simulink model "IP_with_error"  (R2016b)
settings: Solver=FixedStepAuto  StartTime=0.0  StopTime=100  RelTol=1e-3  EnableMultiTasking=on
values from neighbouring files (symbols this model uses):
  A = [0 0 1 0 ... (first row only)    [Controller_IP_with_error.m]    (also in Controller_IP_without_error.m)
  B = [0;0;1;3]    [Controller_IP_with_error.m]    (also in Controller_IP_without_error.m)
  Bw = [0.0015;0.007;0.075;0.35]    [Controller_IP_with_error.m]    (also in Controller_IP_without_error.m)
  K = Ymat*inv(Xmat)    [Controller_IP_with_error.m]    (also in Controller_IP_without_error.m)
settings Model: Creator=Li  LastModifiedBy=silen
settings DataIOCC: LimitDataPoints=on  SaveFormat=Array
settings OptimizationCC: LifeSpan=inf
settings DebuggingCC: SolverPrmCheckMsg=warning  SFUnexpectedBacktrackingDiag=warning  SFNoUnconditionalDefaultTransitionDiag=warning  SFExecutionAtInitializationDiag=none
settings HardwareCC: ProdBitPerPointer=32  ProdBitPerSizeT=32  ProdBitPerPtrDiffT=32  ProdLargestAtomicFloat=None  ProdIntDivRoundTo=Undefined  ProdEndianess=Unspecified  ProdWordSize=32  ProdHWDeviceType=32-bit Generic
settings ModelReferenceCC: PropagateSignalLabelsOutOfModel=off
settings GRTTargetCC: TargetLangStandard=C89/C90 (ANSI)  GeneratePreprocessorConditionals=Disable all
settings ConfigComp: CovMetricSettings=dw  CovHtmlReporting=on  CovSaveCumulativeToWorkspaceVar=on  CovSaveSingleToWorkspaceVar=on  CovExternalEMLEnable=off  CovSFcnEnable=off

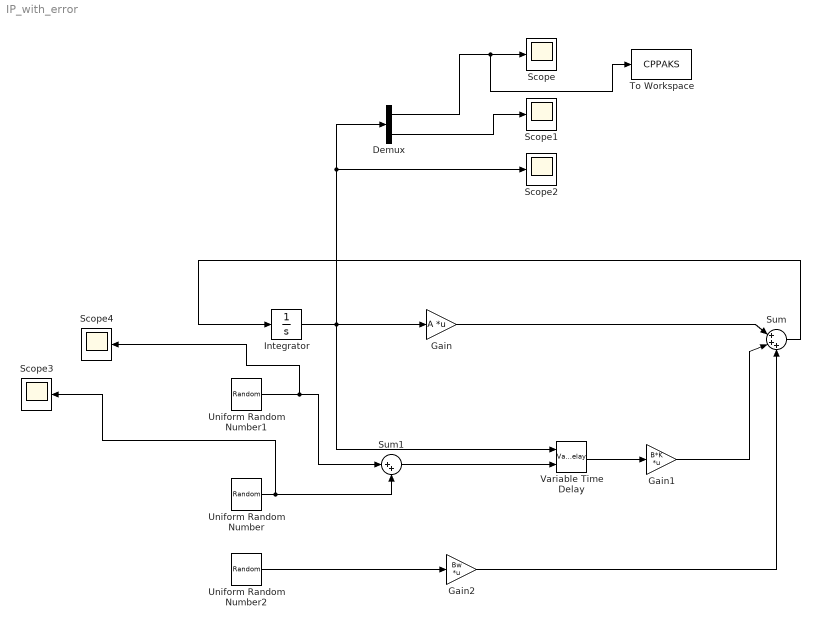
== system IP_with_error ==
  Demux : Demux  Outputs=2
  Gain : Gain  Gain=A  Multiplication=Matrix(K*u)
  Gain1 : Gain  Gain=B*K  Multiplication=Matrix(K*u)
  Gain2 : Gain  Gain=Bw  Multiplication=Matrix(K*u)
  Integrator : Integrator  InitialCondition=[0;0.1;0;0]
  Scope{,1..4} (5 alike) : Scope
  Sum : Sum  Inputs=|+++
  Sum1 : Sum  Inputs=|++
  To Workspace : ToWorkspace  VariableName=CPPAKS  SaveFormat=Timeseries  SampleTime=-1
  Uniform Random Number : UniformRandomNumber  Minimum=0.019  Maximum=0.058  SampleTime=0.1
  Uniform Random Number1 : UniformRandomNumber  Minimum=0  Maximum=0.016  SampleTime=0.1
  Uniform Random Number2 : UniformRandomNumber  SampleTime=0.1
  Variable Time Delay : VariableTransportDelay  MaximumDelay=10
  wires:
  Integrator/1 -> Scope2/1, Demux/1, Variable Time Delay/1, Gain/1
  Gain/1 -> Sum/1
  Gain1/1 -> Sum/2
  Uniform Random Number/1 -> Sum1/2, Scope3/1
  Sum/1 -> Integrator/1
  Demux/1 -> To Workspace/1, Scope/1
  Demux/2 -> Scope1/1
  Uniform Random Number1/1 -> Sum1/1, Scope4/1
  Variable Time Delay/1 -> Gain1/1
  Sum1/1 -> Variable Time Delay/2
  Uniform Random Number2/1 -> Gain2/1
  Gain2/1 -> Sum/3
